simulink model "DvrSimKeybdGD_cs_old"  (R2016a)
settings: Solver=ode5  SolverMode=SingleTasking  StartTime=0.0  StopTime=inf  FixedStep=1/1000  RelTol=1e-3
PreLoadFcn:
  | mbxruntime.callbacks.PreLoadFcn(bdroot);
PostLoadFcn:
  | mbxruntime.callbacks.PostLoadFcn(bdroot);
InitFcn:
  | mbxruntime.callbacks.InitFcn(bdroot);
StartFcn:
  | mbxruntime.callbacks.StartFcn(bdroot);
StopFcn:
  | mbxruntime.callbacks.StopFcn(bdroot);
model workspace (MAT data in the model file):
  mbox_table : struct (value not decoded)
  model_closed = 0
  sim_status = 0
undefined symbols (not defined in the file or in its folder): BMotor1, BMotor2, BrkDelayTime, DControlB, Delay1, Delay2, DiscIntNeverNeededParam, IControlB, JMotor1, JMotor2, PControlB, PreScanCarSimLoadFcn, ratioGearF, ratioGearR, TorqDelayTime, Tstep
undefined symbols (not defined in the file): SteeringColumn, SteeringWheel, WheelL0, WheelL1, WheelR0, WheelR1
libraries: PreScanSimulinkLibrary x35, simulink_extras x26, simulink x26, MyLib x3, Solver_SF x2, pil_lib x1, PreScanUsefulBlocks x1
(part 7 of 12)

== system DvrSimKeybdGD_cs_old/Roewe_550_S_Sedan_1/LaneMarkerSensor_4_Data/If Action Subsystem3 ==
  In1 : Inport
  In2 : Inport  Port=2
  Action Port : ActionPort  ActionType=then
  Bus Selector : BusSelector  OutputSignals=DATA
  Selector : Selector  IndexOptions=Index vector (port)  Indices=[4]  OutputSizes=1
  Out1 : Outport
  wires:
  Bus Selector/1 -> Out1/1  "<DATA>"
  Selector/1 -> Bus Selector/1
  In1/1 -> Selector/1
  In2/1 -> Selector/2

== system DvrSimKeybdGD_cs_old/Roewe_550_S_Sedan_1/LaneMarkerSensor_4_Data/If Action Subsystem4 ==
  In1 : Inport
  In2 : Inport  Port=2
  Action Port : ActionPort  ActionType=then
  Bus Selector : BusSelector  OutputSignals=DATA
  Selector : Selector  IndexOptions=Index vector (port)  Indices=[4]  OutputSizes=1
  Out1 : Outport
  wires:
  Bus Selector/1 -> Out1/1  "<DATA>"
  Selector/1 -> Bus Selector/1
  In1/1 -> Selector/1
  In2/1 -> Selector/2

== system DvrSimKeybdGD_cs_old/Roewe_550_S_Sedan_1/LaneMarkerSensor_5_Data/If Action Subsystem1 ==
  In1 : Inport
  In2 : Inport  Port=2
  Action Port : ActionPort  ActionType=then
  Bus Selector : BusSelector  OutputSignals=DATA
  Selector : Selector  IndexOptions=Index vector (port)  Indices=[4]  OutputSizes=1
  Out1 : Outport
  wires:
  Bus Selector/1 -> Out1/1  "<DATA>"
  Selector/1 -> Bus Selector/1
  In1/1 -> Selector/1
  In2/1 -> Selector/2

== system DvrSimKeybdGD_cs_old/Roewe_550_S_Sedan_1/LaneMarkerSensor_5_Data/If Action Subsystem2 ==
  In1 : Inport
  In2 : Inport  Port=2
  Action Port : ActionPort  ActionType=then
  Bus Selector : BusSelector  OutputSignals=DATA
  Selector : Selector  IndexOptions=Index vector (port)  Indices=[4]  OutputSizes=1
  Out1 : Outport
  wires:
  Bus Selector/1 -> Out1/1  "<DATA>"
  Selector/1 -> Bus Selector/1
  In1/1 -> Selector/1
  In2/1 -> Selector/2

== system DvrSimKeybdGD_cs_old/Roewe_550_S_Sedan_1/LaneMarkerSensor_5_Data/If Action Subsystem3 ==
  In1 : Inport
  In2 : Inport  Port=2
  Action Port : ActionPort  ActionType=then
  Bus Selector : BusSelector  OutputSignals=DATA
  Selector : Selector  IndexOptions=Index vector (port)  Indices=[4]  OutputSizes=1
  Out1 : Outport
  wires:
  Bus Selector/1 -> Out1/1  "<DATA>"
  Selector/1 -> Bus Selector/1
  In1/1 -> Selector/1
  In2/1 -> Selector/2

== system DvrSimKeybdGD_cs_old/Roewe_550_S_Sedan_1/LaneMarkerSensor_5_Data/If Action Subsystem4 ==
  In1 : Inport
  In2 : Inport  Port=2
  Action Port : ActionPort  ActionType=then
  Bus Selector : BusSelector  OutputSignals=DATA
  Selector : Selector  IndexOptions=Index vector (port)  Indices=[4]  OutputSizes=1
  Out1 : Outport
  wires:
  Bus Selector/1 -> Out1/1  "<DATA>"
  Selector/1 -> Bus Selector/1
  In1/1 -> Selector/1
  In2/1 -> Selector/2

== system DvrSimKeybdGD_cs_old/Roewe_550_S_Sedan_1/PreScan_RayCast_Contact_Sensor/Contact Point Bus Creator ==
  demux in : Inport
  Bus Creator : BusCreator  Inputs=3
  Bus Creator1 : BusCreator  Inputs=3
  Bus Creator2 : BusCreator  Inputs=3
  Demux : Demux  Outputs=3
  Demux5 : Demux  Outputs=[3 3 1]
  Demux6 : Demux  Outputs=3
  bus out : Outport
  wires:
  Demux/1 -> Bus Creator/1  "x"
  Demux/2 -> Bus Creator/2  "y"
  Demux/3 -> Bus Creator/3  "z"
  Demux6/1 -> Bus Creator1/1  "x"
  Demux6/2 -> Bus Creator1/2  "y"
  Demux6/3 -> Bus Creator1/3  "z"
  demux in/1 -> Demux5/1
  Demux5/3 -> Bus Creator2/3  "penetrationdepth"
  Bus Creator2/1 -> bus out/1
  Demux5/1 -> Demux/1
  Demux5/2 -> Demux6/1
  Bus Creator/1 -> Bus Creator2/1  "normal"
  Bus Creator1/1 -> Bus Creator2/2  "position"

== system DvrSimKeybdGD_cs_old/Roewe_550_S_Sedan_1/PreScan_RayCast_Contact_Sensor/Contact Point Bus Creator1 ==
  demux in : Inport
  Bus Creator : BusCreator  Inputs=3
  Bus Creator1 : BusCreator  Inputs=3
  Bus Creator2 : BusCreator  Inputs=3
  Demux : Demux  Outputs=3
  Demux5 : Demux  Outputs=[3 3 1]
  Demux6 : Demux  Outputs=3
  bus out : Outport
  wires:
  Bus Creator1/1 -> Bus Creator2/2  "position"
  Bus Creator/1 -> Bus Creator2/1  "normal"
  Demux5/2 -> Demux6/1
  Demux5/1 -> Demux/1
  Bus Creator2/1 -> bus out/1
  Demux5/3 -> Bus Creator2/3  "penetrationdepth"
  demux in/1 -> Demux5/1
  Demux6/3 -> Bus Creator1/3  "z"
  Demux6/2 -> Bus Creator1/2  "y"
  Demux6/1 -> Bus Creator1/1  "x"
  Demux/3 -> Bus Creator/3  "z"
  Demux/2 -> Bus Creator/2  "y"
  Demux/1 -> Bus Creator/1  "x"

== system DvrSimKeybdGD_cs_old/Roewe_550_S_Sedan_1/PreScan_RayCast_Contact_Sensor/Contact Point Bus Creator2 ==
  demux in : Inport
  Bus Creator : BusCreator  Inputs=3
  Bus Creator1 : BusCreator  Inputs=3
  Bus Creator2 : BusCreator  Inputs=3
  Demux : Demux  Outputs=3
  Demux5 : Demux  Outputs=[3 3 1]
  Demux6 : Demux  Outputs=3
  bus out : Outport
  wires:
  Bus Creator1/1 -> Bus Creator2/2  "position"
  Bus Creator/1 -> Bus Creator2/1  "normal"
  Demux5/2 -> Demux6/1
  Demux5/1 -> Demux/1
  Bus Creator2/1 -> bus out/1
  Demux5/3 -> Bus Creator2/3  "penetrationdepth"
  demux in/1 -> Demux5/1
  Demux6/3 -> Bus Creator1/3  "z"
  Demux6/2 -> Bus Creator1/2  "y"
  Demux6/1 -> Bus Creator1/1  "x"
  Demux/3 -> Bus Creator/3  "z"
  Demux/2 -> Bus Creator/2  "y"
  Demux/1 -> Bus Creator/1  "x"

== system DvrSimKeybdGD_cs_old/Roewe_550_S_Sedan_1/PreScan_RayCast_Contact_Sensor/Contact Point Bus Creator3 ==
  demux in : Inport
  Bus Creator : BusCreator  Inputs=3
  Bus Creator1 : BusCreator  Inputs=3
  Bus Creator2 : BusCreator  Inputs=3
  Demux : Demux  Outputs=3
  Demux5 : Demux  Outputs=[3 3 1]
  Demux6 : Demux  Outputs=3
  bus out : Outport
  wires:
  Bus Creator1/1 -> Bus Creator2/2  "position"
  Bus Creator/1 -> Bus Creator2/1  "normal"
  Demux5/2 -> Demux6/1
  Demux5/1 -> Demux/1
  Bus Creator2/1 -> bus out/1
  Demux5/3 -> Bus Creator2/3  "penetrationdepth"
  demux in/1 -> Demux5/1
  Demux6/3 -> Bus Creator1/3  "z"
  Demux6/2 -> Bus Creator1/2  "y"
  Demux6/1 -> Bus Creator1/1  "x"
  Demux/3 -> Bus Creator/3  "z"
  Demux/2 -> Bus Creator/2  "y"
  Demux/1 -> Bus Creator/1  "x"

== system DvrSimKeybdGD_cs_old/Roewe_550_S_Sedan_1/PreScan_RayCast_Contact_Sensor/For All Wheel Contacts ==
  In1 : Inport  Partition=on  PartitionDimension=1  PartitionWidth=1
  Bus Selector : BusSelector  OutputSignals=NORMAL.X,NORMAL.Y,NORMAL.Z,POSITION.X,POSITION.Y,POSITION.Z,PENETRATIONDEPTH
  For Each : ForEach  DisableCoverage=on  IndexMode=One-based
  Mux : Mux  Inputs=7
  Out1 : Outport  ConcatenationDimension=1
  wires:
  In1/1 -> Bus Selector/1
  Bus Selector/1 -> Mux/1  "<X>"
  Bus Selector/2 -> Mux/2  "<Y>"
  Bus Selector/3 -> Mux/3  "<Z>"
  Bus Selector/4 -> Mux/4  "<X>"
  Bus Selector/5 -> Mux/5  "<Y>"
  Bus Selector/6 -> Mux/6  "<Z>"
  Bus Selector/7 -> Mux/7  "<PENETRATIONDEPTH>"
  Mux/1 -> Out1/1

== system DvrSimKeybdGD_cs_old/Roewe_550_S_Sedan_1/PreScan_RayCast_Contact_Sensor/Subsystem1 ==
  In1 : Inport
  sfun_WheelContactsRayCast : S-Function  FunctionName=sfun_WheelContactsRayCast  Parameters=SParameter1, SParameter2, SParameter3, SParameter4, SParameter5, SampleTime  SFunctionDeploymentMode=off  EnableBusSupport=off  mask(Legacy Function){SFunctionSpec=void prescan_outputFcn(void ** work1,  PRESCAN_POSEQ_DATA u1[p3], PRESCAN_WHEELCONTACT_DATA y1[p4]), SParameter1=uint8([fullfile(pwd,'Experiment.pex') 0]), SParameter2=uint8([0 0]), SParameter3=NumberOfWheels, SParameter4=NumberOfWheels*MaxContactPoints, SParameter5=Range, SampleTime=-1, ShowSpec=on}
      mask prompts: SParameter1 "P1:"; SParameter2 "P2:"; SParameter3 "P3:"; SParameter4 "P4:"; SParameter5 "P5:"; SampleTime "Sample time (-1 for inherited):"; ShowSpec "Display function specification"
      mask help:
      | This block allows you to call the legacy functions specified by the following Legacy Code Tool definition:
      | def.SFunctionName = 'sfun_WheelContactsRayCast';
      | def.OutputFcnSpec = 'void prescan_outputFcn(void ** work1,  PRESCAN_POSEQ_DATA u1[p3], PRESCAN_WHEELCONTACT_DATA y1[p4])';
      | def.StartFcnSpec = 'void prescan_startFcn(void ** work1, uint8 p1[], uint8 p2[], double p3, double p4, double p5)';
      | def.TerminateFcnSpec = 'void prescan_terminateFcn(void ** work1)';
      | def.HeaderFiles = {'prescan_wheelcontactsraycast_data.h', 'prescan_header_data.h', 'prescan_SFunLibrary.h', 'prescan_CreateLogHandler.h', 'prescan_CreateErrorHandler.h'};
      | def.SourceFiles = {'prescan_MexLogHandler.cpp', 'prescan_SimStructErrorHandler.cpp', 'prescan_ConcurrentLogHandler.cpp', 'prescan_ConcurrentErrorHandler.cpp'};
      | def.HostLibFiles = {'sensorinterfaced.lib'};
      | def.TargetLibFiles = {'sensorinterfaced.so'};
      | def.IncPaths = {'.', 'C:\prescandev\vislibrary\vis\..\pimp\include\sensors\InterfaceRTW'};
      | def.SrcPaths = {'.'};
      | def.LibPaths = {'C:\\prescandev\\vislibrary_build\lib'};
      | def.SampleTime = 'parameterized';
      mask Help: <p>This block was generated automatically by the Legacy Code Tool. For detailed help on this tool, call<a href="matlab:legacy_code('help')"> legacy_code('help')</a>.</p>
      mask Callback ShowSpec:
      | if strcmp(get_param(gcbh, 'ShowSpec'), 'on')
      |   set_param(gcbh, 'MaskDisplay', sprintf('fprintf(''%s'');', get_param(gcbh, 'SFunctionSpec')));
      | else
      |   set_param(gcbh, 'MaskDisplay', sprintf('fprintf(''%s'');', get_param(gcbh, 'FunctionName')));
      | end
      mask Display: fprintf('void prescan_outputFcn(void ** work1,  PRESCAN_POSEQ_DATA u1[p3], PRESCAN_WHEELCONTACT_DATA y1[p4])');
  Out1 : Outport
  wires:
  In1/1 -> sfun_WheelContactsRayCast/1
  sfun_WheelContactsRayCast/1 -> Out1/1

== system DvrSimKeybdGD_cs_old/Roewe_550_S_Sedan_1/PreScan_RayCast_Contact_Sensor/Subsystem2 ==
  Wheel poses : Inport
  Wheel radius : Inport  Port=2
  Vehicle orientation : Inport  Port=3
  Bus Creator : BusCreator  Inputs=3
  Demux3 : Demux  Outputs=3
  sfun_WheelPoseCorrection : S-Function  FunctionName=sfun_WheelPoseCorrection  Parameters=SParameter1, SampleTime  SFunctionDeploymentMode=off  EnableBusSupport=off  mask(Legacy Function){SFunctionSpec=void prescan_outputFcn(void ** work1,  PRESCAN_POSEQ_DATA u1[p1], double u2[p1], PRESCAN_RPY_DATA u3[1], PRESCAN_POSEQ_DATA y1[p1]), SParameter1=nrOfWheels, SampleTime=-1, ShowSpec=on}
      mask prompts: SParameter1 "P1:"; SampleTime "Sample time (-1 for inherited):"; ShowSpec "Display function specification"
      mask help:
      | This block allows you to call the legacy functions specified by the following Legacy Code Tool definition:
      | def.SFunctionName = 'sfun_WheelPoseCorrection';
      | def.OutputFcnSpec = 'void prescan_outputFcn(void ** work1,  PRESCAN_POSEQ_DATA u1[p1], double u2[p1], PRESCAN_RPY_DATA u3[1], PRESCAN_POSEQ_DATA y1[p1])';
      | def.StartFcnSpec = 'void prescan_startFcn(void ** work1, double p1)';
      | def.TerminateFcnSpec = 'void prescan_terminateFcn(void ** work1)';
      | def.HeaderFiles = {'prescan_wheelposecorrection_data.h', 'prescan_header_data.h', 'prescan_SFunLibrary.h', 'prescan_CreateLogHandler.h', 'prescan_CreateErrorHandler.h'};
      | def.SourceFiles = {'prescan_MexLogHandler.cpp', 'prescan_SimStructErrorHandler.cpp', 'prescan_ConcurrentLogHandler.cpp', 'prescan_ConcurrentErrorHandler.cpp'};
      | def.HostLibFiles = {'sensorinterfaced.lib'};
      | def.TargetLibFiles = {'sensorinterfaced.so'};
      | def.IncPaths = {'.', 'C:\prescandev\vislibrary\vis\..\pimp\include\sensors\InterfaceRTW'};
      | def.SrcPaths = {'.'};
      | def.LibPaths = {'C:\\prescandev\\vislibrary_build\lib'};
      | def.SampleTime = 'parameterized';
      mask Help: <p>This block was generated automatically by the Legacy Code Tool. For detailed help on this tool, call<a href="matlab:legacy_code('help')"> legacy_code('help')</a>.</p>
      mask Callback ShowSpec:
      | if strcmp(get_param(gcbh, 'ShowSpec'), 'on')
      |   set_param(gcbh, 'MaskDisplay', sprintf('fprintf(''%s'');', get_param(gcbh, 'SFunctionSpec')));
      | else
      |   set_param(gcbh, 'MaskDisplay', sprintf('fprintf(''%s'');', get_param(gcbh, 'FunctionName')));
      | end
      mask Display: fprintf('void prescan_outputFcn(void ** work1,  PRESCAN_POSEQ_DATA u1[p1], double u2[p1], PRESCAN_RPY_DATA u3[1], PRESCAN_POSEQ_DATA y1[p1])');
  Virtual Poses : Outport
  wires:
  Demux3/1 -> Bus Creator/1  "Roll"
  Demux3/2 -> Bus Creator/2  "Pitch"
  Demux3/3 -> Bus Creator/3  "Yaw"
  Bus Creator/1 -> sfun_WheelPoseCorrection/3
  Wheel radius/1 -> sfun_WheelPoseCorrection/2
  Vehicle orientation/1 -> Demux3/1
  sfun_WheelPoseCorrection/1 -> Virtual Poses/1
  Wheel poses/1 -> sfun_WheelPoseCorrection/1

== system DvrSimKeybdGD_cs_old/Roewe_550_S_Sedan_1/PreScan_RayCast_Contact_Sensor/Vehicle Local to World ==
  State : Inport
  Demux1 : Demux  Outputs=[3 3]
  iniBODYAngles wrtVEH [rad] : Constant  Value=[Roll0 Pitch0 0]  SampleTime=Inf
  iniVEHAngles wrtGLOB [rad] : Constant  Value=[0 0 Yaw0]  SampleTime=Inf
  iniVEHposition wrtGLOB [m] : Constant  Value=[x0 y0 z0]  SampleTime=Inf
  state2FullState : Subsystem  mask(PreScan Demux Block:){}
  Position : Outport
  Orientation : Outport  Port=2
  wires:
  iniVEHAngles wrtGLOB [rad]/1 -> state2FullState/4(iniVEH Angles wrt GLOB axis system [deg])
  iniBODYAngles wrtVEH [rad]/1 -> state2FullState/3(iniBODY Angles wrt VEH axis system [deg])
  iniVEHposition wrtGLOB [m]/1 -> state2FullState/2(ini VEHpos wrt GLOB axis system [m])
  Demux1/2 -> Orientation/1
  Demux1/1 -> Position/1
  State/1 -> state2FullState/1(dx,dy,dz [m/s] R,P,Y [rad])
  state2FullState/1(State) -> Demux1/1

== system DvrSimKeybdGD_cs_old/Roewe_550_S_Sedan_1/PreScan_RayCast_Contact_Sensor/Wheels = 4 ==
  Vehicle wrt World : Inport
  Wheels wrt World : Inport  Port=2
  Bus Creator : BusCreator  Inputs=3  OutDataTypeStr=Bus: PRESCAN_XYZ_DATA  NonVirtualBus=on
  Bus Creator1 : BusCreator  Inputs=3  OutDataTypeStr=Bus: PRESCAN_RPY_DATA  NonVirtualBus=on
  Bus Creator3 : BusCreator  Inputs=2  OutDataTypeStr=Bus: PRESCAN_POSE_DATA  NonVirtualBus=on
  Demux3 : Demux  Outputs=6
  FL : Selector  InputPortWidth=28  IndexOptions=Index vector (dialog)  Indices=[(1:7)]  OutputSizes=1
  FR : Selector  InputPortWidth=28  IndexOptions=Index vector (dialog)  Indices=[(8:14)]  OutputSizes=1
  RL : Selector  InputPortWidth=28  IndexOptions=Index vector (dialog)  Indices=[(15:21)]  OutputSizes=1
  RR : Selector  InputPortWidth=28  IndexOptions=Index vector (dialog)  Indices=[(22:28)]  OutputSizes=1
  Vector Concatenate1 : Concatenate  NumInputs=4
  sfun_Wheels2World : S-Function  FunctionName=sfun_Wheels2World  Parameters=SParameter1, SParameter2, SParameter3, SampleTime  SFunctionDeploymentMode=off  EnableBusSupport=off  mask(Legacy Function){SFunctionSpec=void prescan_outputFcn(void ** work1,  PRESCAN_POSE_DATA u1[1], PRESCAN_POSEA_DATA u2[p1], PRESCAN_POSEQ_DATA y1[p1]), SParameter1=NumberOfWheels, SParameter2=hcog, SParameter3=b, SampleTime=-1, ShowSpec=on}
      mask prompts: SParameter1 "P1:"; SParameter2 "P2:"; SParameter3 "P3:"; SampleTime "Sample time (-1 for inherited):"; ShowSpec "Display function specification"
      mask help:
      | This block allows you to call the legacy functions specified by the following Legacy Code Tool definition:
      | def.SFunctionName = 'sfun_Wheels2World';
      | def.OutputFcnSpec = 'void prescan_outputFcn(void ** work1,  PRESCAN_POSE_DATA u1[1], PRESCAN_POSEA_DATA u2[p1], PRESCAN_POSEQ_DATA y1[p1])';
      | def.StartFcnSpec = 'void prescan_startFcn(void ** work1, double p1, double p2, double p3)';
      | def.TerminateFcnSpec = 'void prescan_terminateFcn(void ** work1)';
      | def.HeaderFiles = {'prescan_wheels2world_data.h', 'prescan_header_data.h', 'prescan_SFunLibrary.h', 'prescan_CreateLogHandler.h', 'prescan_CreateErrorHandler.h'};
      | def.SourceFiles = {'prescan_MexLogHandler.cpp', 'prescan_SimStructErrorHandler.cpp', 'prescan_ConcurrentLogHandler.cpp', 'prescan_ConcurrentErrorHandler.cpp'};
      | def.HostLibFiles = {'sensorinterfaced.lib'};
      | def.TargetLibFiles = {'sensorinterfaced.so'};
      | def.IncPaths = {'.', 'C:\prescandev\vislibrary\vis\..\pimp\include\sensors\InterfaceRTW'};
      | def.SrcPaths = {'.'};
      | def.LibPaths = {'C:\\prescandev\\vislibrary_build\lib'};
      | def.SampleTime = 'parameterized';
      mask Help: <p>This block was generated automatically by the Legacy Code Tool. For detailed help on this tool, call<a href="matlab:legacy_code('help')"> legacy_code('help')</a>.</p>
      mask Callback ShowSpec:
      | if strcmp(get_param(gcbh, 'ShowSpec'), 'on')
      |   set_param(gcbh, 'MaskDisplay', sprintf('fprintf(''%s'');', get_param(gcbh, 'SFunctionSpec')));
      | else
      |   set_param(gcbh, 'MaskDisplay', sprintf('fprintf(''%s'');', get_param(gcbh, 'FunctionName')));
      | end
      mask Display: fprintf('void prescan_outputFcn(void ** work1,  PRESCAN_POSE_DATA u1[1], PRESCAN_POSEA_DATA u2[p1], PRESCAN_POSEQ_DATA y1[p1])');
  wheelposeFL : Subsystem
  wheelposeFR : Subsystem
  wheelposeRL : Subsystem
  wheelposeRR : Subsystem
  WheelPoses : Outport
  wires:
  FL/1 -> wheelposeFL/1(vector)
  FR/1 -> wheelposeFR/1(vector)
  RL/1 -> wheelposeRL/1(vector)
  RR/1 -> wheelposeRR/1(vector)
  wheelposeFL/1(bus) -> Vector Concatenate1/1
  Demux3/1 -> Bus Creator/1  "X"
  Demux3/2 -> Bus Creator/2  "Y"
  Demux3/3 -> Bus Creator/3  "Z"
  Demux3/4 -> Bus Creator1/1  "Roll"
  Demux3/5 -> Bus Creator1/2  "Pitch"
  Demux3/6 -> Bus Creator1/3  "Yaw"
  Bus Creator/1 -> Bus Creator3/1  "POSITION"
  Bus Creator1/1 -> Bus Creator3/2  "ORIENTATION"
  Vehicle wrt World/1 -> Demux3/1
  Wheels wrt World/1 -> FL/1, FR/1, RL/1, RR/1
  sfun_Wheels2World/1 -> WheelPoses/1
  wheelposeFR/1(bus) -> Vector Concatenate1/2
  wheelposeRL/1(bus) -> Vector Concatenate1/3
  wheelposeRR/1(bus) -> Vector Concatenate1/4
  Bus Creator3/1 -> sfun_Wheels2World/1
  Vector Concatenate1/1 -> sfun_Wheels2World/2

== system DvrSimKeybdGD_cs_old/Roewe_550_S_Sedan_1/PreScan_RayCast_Contact_Sensor/Wheels Local to World ==
  Steer Angle Front [deg] : Inport  SampleTime=TimeStep
  Steer Angle Rear [deg] : Inport  Port=2  SampleTime=TimeStep
  Velocity [m/s] : Inport  Port=3  SampleTime=TimeStep
  Disp FL [m] : Inport  Port=4  SampleTime=TimeStep
  Disp FR [m] : Inport  Port=5  SampleTime=TimeStep
  Disp RL [m] : Inport  Port=6  SampleTime=TimeStep
  Disp RR [m] : Inport  Port=7  SampleTime=TimeStep
  Constant{4..7} (4 alike) : Constant  Value=0  SampleTime=Inf
  Discrete-Time Integrator : DiscreteIntegrator  SampleTime=TimeStep  ICPrevOutput=DiscIntNeverNeededParam  ICPrevScaledInput=DiscIntNeverNeededParam
  Mux{,1..3} (4 alike) : Mux  Inputs=3
  Mux5 : Mux  Inputs=[3 4 3 4 3 4 3 4]
  Radians to Degrees : simulink_extras/Transformations/Radians to Degrees
  Saturation{,2,4,6} (4 alike) : Saturate  UpperLimit=[0.2 0.2 0.5]  LowerLimit=[-0.2 -0.2 -0.5]
  Saturation{1,3,5,8} (4 alike) : Saturate  UpperLimit=[30 inf 30]  LowerLimit=[-30 -inf -30]
  conv_RotWheelFL : Subsystem
  conv_RotWheelFR : Subsystem
  conv_RotWheelRL : Subsystem
  conv_RotWheelRR : Subsystem
  conv_TransWheelFL : Subsystem  mask(Translation node configuration){tp=Front-Left Wheel, gains=off, Gain_xISO=1, Gain_yISO=1, Gain_zISO=1}
      mask prompts: tp "Type"; gains "Edit scaling factors?"; Gain_xISO "Scaling factor in x-direction (ISO-convention)"; Gain_yISO "Scaling factor in y-direction (ISO-convention)"; Gain_zISO "Scaling factor in z-direction (ISO-convention)"
      mask init:
      | x_ini_VRML = 2.701790; 
      | y_ini_VRML = 0.665750; 
      | z_ini_VRML = 0.317714;
      mask TypeOptions tp: Front-Left Wheel | Front-Right Wheel | Rear-Left Wheel | Rear-Right Wheel | Left Seat | Right Seat
      mask Callback gains:
      | if strcmp(get_param(gcb, 'gains'),'on')
      |     set_param(gcb,'MaskVisibilities',{'on','on','on','on','on'})
      | else
      |     set_param(gcb,'MaskVisibilities',{'on','on','off','off','off'})
      | end
  conv_TransWheelFR : Subsystem  mask(Translation node configuration){tp=Front-Right Wheel, gains=off, Gain_xISO=1, Gain_yISO=1, Gain_zISO=1}
      mask prompts: tp "Type"; gains "Edit scaling factors?"; Gain_xISO "Scaling factor in x-direction (ISO-convention)"; Gain_yISO "Scaling factor in y-direction (ISO-convention)"; Gain_zISO "Scaling factor in z-direction (ISO-convention)"
      mask init:
      | x_ini_VRML = 2.701790; 
      | y_ini_VRML = -0.665750; 
      | z_ini_VRML = 0.317714;
      mask TypeOptions tp: Front-Left Wheel | Front-Right Wheel | Rear-Left Wheel | Rear-Right Wheel | Left Seat | Right Seat
      mask Callback gains:
      | if strcmp(get_param(gcb, 'gains'),'on')
      |     set_param(gcb,'MaskVisibilities',{'on','on','on','on','on'})
      | else
      |     set_param(gcb,'MaskVisibilities',{'on','on','off','off','off'})
      | end
  conv_TransWheelRL : Subsystem  mask(Translation node configuration){tp=Rear-Left Wheel, gains=off, Gain_xISO=1, Gain_yISO=1, Gain_zISO=1}
      mask prompts: tp "Type"; gains "Edit scaling factors?"; Gain_xISO "Scaling factor in x-direction (ISO-convention)"; Gain_yISO "Scaling factor in y-direction (ISO-convention)"; Gain_zISO "Scaling factor in z-direction (ISO-convention)"
      mask init:
      | x_ini_VRML = 0.000000; 
      | y_ini_VRML = 0.665750; 
      | z_ini_VRML = 0.317714;
      mask TypeOptions tp: Front-Left Wheel | Front-Right Wheel | Rear-Left Wheel | Rear-Right Wheel | Left Seat | Right Seat
      mask Callback gains:
      | if strcmp(get_param(gcb, 'gains'),'on')
      |     set_param(gcb,'MaskVisibilities',{'on','on','on','on','on'})
      | else
      |     set_param(gcb,'MaskVisibilities',{'on','on','off','off','off'})
      | end
  conv_TransWheelRR : Subsystem  mask(Translation node configuration){tp=Rear-Right Wheel, gains=off, Gain_xISO=1, Gain_yISO=1, Gain_zISO=1}
      mask prompts: tp "Type"; gains "Edit scaling factors?"; Gain_xISO "Scaling factor in x-direction (ISO-convention)"; Gain_yISO "Scaling factor in y-direction (ISO-convention)"; Gain_zISO "Scaling factor in z-direction (ISO-convention)"
      mask init:
      | x_ini_VRML = 0.000000; 
      | y_ini_VRML = -0.665750; 
      | z_ini_VRML = 0.317714;
      mask TypeOptions tp: Front-Left Wheel | Front-Right Wheel | Rear-Left Wheel | Rear-Right Wheel | Left Seat | Right Seat
      mask Callback gains:
      | if strcmp(get_param(gcb, 'gains'),'on')
      |     set_param(gcb,'MaskVisibilities',{'on','on','on','on','on'})
      | else
      |     set_param(gcb,'MaskVisibilities',{'on','on','off','off','off'})
      | end
  omega=V/Rwheel : Gain  Gain=1/0.29
  Wheel Poses : Outport
  wires:
  conv_RotWheelRR/1(QuaternionVisu [rad]) -> Mux5/8
  conv_RotWheelRL/1(QuaternionVisu [rad]) -> Mux5/6
  conv_TransWheelRR/1(transVisu [m]) -> Mux5/7
  conv_TransWheelRL/1(transVisu [m]) -> Mux5/5
  conv_RotWheelFR/1(QuaternionVisu [rad]) -> Mux5/4
  conv_TransWheelFR/1(transVisu [m]) -> Mux5/3
  conv_RotWheelFL/1(QuaternionVisu [rad]) -> Mux5/2
  conv_TransWheelFL/1(transVisu [m]) -> Mux5/1
  Saturation/1 -> conv_TransWheelFL/1(transISO [m])
  Saturation8/1 -> conv_RotWheelFL/1(BryantISO [deg])
  Saturation2/1 -> conv_TransWheelFR/1(transISO [m])
  Saturation1/1 -> conv_RotWheelFR/1(BryantISO [deg])
  Saturation4/1 -> conv_TransWheelRL/1(transISO [m])
  Saturation3/1 -> conv_RotWheelRL/1(BryantISO [deg])
  Saturation6/1 -> conv_TransWheelRR/1(transISO [m])
  Saturation5/1 -> conv_RotWheelRR/1(BryantISO [deg])
  Mux5/1 -> Wheel Poses/1
  Mux2/1 -> Saturation3/1  "xyz rotation RL [deg]"
  Mux3/1 -> Saturation5/1  "xyz rotation RR [deg]"
  Mux/1 -> Saturation8/1  "xyz rotation FL [deg]"
  Mux1/1 -> Saturation1/1  "xyz rotation FR [deg]"
  Velocity [m/s]/1 -> omega=V/Rwheel/1
  omega=V/Rwheel/1 -> Radians to Degrees/1  "rotational speed [rad/s]"
  Steer Angle Rear [deg]/1 -> Mux2/3, Mux3/3  "rotz"
  Steer Angle Front [deg]/1 -> Mux/3, Mux1/3  "rotz"
  Constant4/1 -> Mux/1  "rotx"
  Constant5/1 -> Mux1/1  "rotx"
  Constant6/1 -> Mux2/1  "rotx"
  Constant7/1 -> Mux3/1  "rotx"
  Radians to Degrees/1 -> Discrete-Time Integrator/1
  Discrete-Time Integrator/1 -> Mux3/2, Mux2/2, Mux1/2, Mux/2  "roty"
  Disp FL [m]/1 -> Saturation/1
  Disp FR [m]/1 -> Saturation2/1
  Disp RL [m]/1 -> Saturation4/1
  Disp RR [m]/1 -> Saturation6/1

== system DvrSimKeybdGD_cs_old/Roewe_550_S_Sedan_1/PreScan_RayCast_Contact_Sensor1/Contact Point Bus Creator ==
  demux in : Inport
  Bus Creator : BusCreator  Inputs=3
  Bus Creator1 : BusCreator  Inputs=3
  Bus Creator2 : BusCreator  Inputs=3
  Demux : Demux  Outputs=3
  Demux5 : Demux  Outputs=[3 3 1]
  Demux6 : Demux  Outputs=3
  bus out : Outport
  wires:
  Demux/1 -> Bus Creator/1  "x"
  Demux/2 -> Bus Creator/2  "y"
  Demux/3 -> Bus Creator/3  "z"
  Demux6/1 -> Bus Creator1/1  "x"
  Demux6/2 -> Bus Creator1/2  "y"
  Demux6/3 -> Bus Creator1/3  "z"
  demux in/1 -> Demux5/1
  Demux5/3 -> Bus Creator2/3  "penetrationdepth"
  Bus Creator2/1 -> bus out/1
  Demux5/1 -> Demux/1
  Demux5/2 -> Demux6/1
  Bus Creator/1 -> Bus Creator2/1  "normal"
  Bus Creator1/1 -> Bus Creator2/2  "position"

== system DvrSimKeybdGD_cs_old/Roewe_550_S_Sedan_1/PreScan_RayCast_Contact_Sensor1/Contact Point Bus Creator1 ==
  demux in : Inport
  Bus Creator : BusCreator  Inputs=3
  Bus Creator1 : BusCreator  Inputs=3
  Bus Creator2 : BusCreator  Inputs=3
  Demux : Demux  Outputs=3
  Demux5 : Demux  Outputs=[3 3 1]
  Demux6 : Demux  Outputs=3
  bus out : Outport
  wires:
  Bus Creator1/1 -> Bus Creator2/2  "position"
  Bus Creator/1 -> Bus Creator2/1  "normal"
  Demux5/2 -> Demux6/1
  Demux5/1 -> Demux/1
  Bus Creator2/1 -> bus out/1
  Demux5/3 -> Bus Creator2/3  "penetrationdepth"
  demux in/1 -> Demux5/1
  Demux6/3 -> Bus Creator1/3  "z"
  Demux6/2 -> Bus Creator1/2  "y"
  Demux6/1 -> Bus Creator1/1  "x"
  Demux/3 -> Bus Creator/3  "z"
  Demux/2 -> Bus Creator/2  "y"
  Demux/1 -> Bus Creator/1  "x"

== system DvrSimKeybdGD_cs_old/Roewe_550_S_Sedan_1/PreScan_RayCast_Contact_Sensor1/Contact Point Bus Creator2 ==
  demux in : Inport
  Bus Creator : BusCreator  Inputs=3
  Bus Creator1 : BusCreator  Inputs=3
  Bus Creator2 : BusCreator  Inputs=3
  Demux : Demux  Outputs=3
  Demux5 : Demux  Outputs=[3 3 1]
  Demux6 : Demux  Outputs=3
  bus out : Outport
  wires:
  Bus Creator1/1 -> Bus Creator2/2  "position"
  Bus Creator/1 -> Bus Creator2/1  "normal"
  Demux5/2 -> Demux6/1
  Demux5/1 -> Demux/1
  Bus Creator2/1 -> bus out/1
  Demux5/3 -> Bus Creator2/3  "penetrationdepth"
  demux in/1 -> Demux5/1
  Demux6/3 -> Bus Creator1/3  "z"
  Demux6/2 -> Bus Creator1/2  "y"
  Demux6/1 -> Bus Creator1/1  "x"
  Demux/3 -> Bus Creator/3  "z"
  Demux/2 -> Bus Creator/2  "y"
  Demux/1 -> Bus Creator/1  "x"

== system DvrSimKeybdGD_cs_old/Roewe_550_S_Sedan_1/PreScan_RayCast_Contact_Sensor1/Contact Point Bus Creator3 ==
  demux in : Inport
  Bus Creator : BusCreator  Inputs=3
  Bus Creator1 : BusCreator  Inputs=3
  Bus Creator2 : BusCreator  Inputs=3
  Demux : Demux  Outputs=3
  Demux5 : Demux  Outputs=[3 3 1]
  Demux6 : Demux  Outputs=3
  bus out : Outport
  wires:
  Bus Creator1/1 -> Bus Creator2/2  "position"
  Bus Creator/1 -> Bus Creator2/1  "normal"
  Demux5/2 -> Demux6/1
  Demux5/1 -> Demux/1
  Bus Creator2/1 -> bus out/1
  Demux5/3 -> Bus Creator2/3  "penetrationdepth"
  demux in/1 -> Demux5/1
  Demux6/3 -> Bus Creator1/3  "z"
  Demux6/2 -> Bus Creator1/2  "y"
  Demux6/1 -> Bus Creator1/1  "x"
  Demux/3 -> Bus Creator/3  "z"
  Demux/2 -> Bus Creator/2  "y"
  Demux/1 -> Bus Creator/1  "x"

== system DvrSimKeybdGD_cs_old/Roewe_550_S_Sedan_1/PreScan_RayCast_Contact_Sensor1/For All Wheel Contacts ==
  In1 : Inport  Partition=on  PartitionDimension=1  PartitionWidth=1
  Bus Selector : BusSelector  OutputSignals=NORMAL.X,NORMAL.Y,NORMAL.Z,POSITION.X,POSITION.Y,POSITION.Z,PENETRATIONDEPTH
  For Each : ForEach  DisableCoverage=on  IndexMode=One-based
  Mux : Mux  Inputs=7
  Out1 : Outport  ConcatenationDimension=1
  wires:
  In1/1 -> Bus Selector/1
  Bus Selector/1 -> Mux/1  "<X>"
  Bus Selector/2 -> Mux/2  "<Y>"
  Bus Selector/3 -> Mux/3  "<Z>"
  Bus Selector/4 -> Mux/4  "<X>"
  Bus Selector/5 -> Mux/5  "<Y>"
  Bus Selector/6 -> Mux/6  "<Z>"
  Bus Selector/7 -> Mux/7  "<PENETRATIONDEPTH>"
  Mux/1 -> Out1/1

== system DvrSimKeybdGD_cs_old/Roewe_550_S_Sedan_1/PreScan_RayCast_Contact_Sensor1/Subsystem1 ==
  In1 : Inport
  sfun_WheelContactsRayCast : S-Function  FunctionName=sfun_WheelContactsRayCast  Parameters=SParameter1, SParameter2, SParameter3, SParameter4, SParameter5, SampleTime  SFunctionDeploymentMode=off  EnableBusSupport=off  mask(Legacy Function){SFunctionSpec=void prescan_outputFcn(void ** work1,  PRESCAN_POSEQ_DATA u1[p3], PRESCAN_WHEELCONTACT_DATA y1[p4]), SParameter1=uint8([fullfile(pwd,'Experiment.pex') 0]), SParameter2=uint8([0 0]), SParameter3=NumberOfWheels, SParameter4=NumberOfWheels*MaxContactPoints, SParameter5=Range, SampleTime=-1, ShowSpec=on}
      mask prompts: SParameter1 "P1:"; SParameter2 "P2:"; SParameter3 "P3:"; SParameter4 "P4:"; SParameter5 "P5:"; SampleTime "Sample time (-1 for inherited):"; ShowSpec "Display function specification"
      mask help:
      | This block allows you to call the legacy functions specified by the following Legacy Code Tool definition:
      | def.SFunctionName = 'sfun_WheelContactsRayCast';
      | def.OutputFcnSpec = 'void prescan_outputFcn(void ** work1,  PRESCAN_POSEQ_DATA u1[p3], PRESCAN_WHEELCONTACT_DATA y1[p4])';
      | def.StartFcnSpec = 'void prescan_startFcn(void ** work1, uint8 p1[], uint8 p2[], double p3, double p4, double p5)';
      | def.TerminateFcnSpec = 'void prescan_terminateFcn(void ** work1)';
      | def.HeaderFiles = {'prescan_wheelcontactsraycast_data.h', 'prescan_header_data.h', 'prescan_SFunLibrary.h', 'prescan_CreateLogHandler.h', 'prescan_CreateErrorHandler.h'};
      | def.SourceFiles = {'prescan_MexLogHandler.cpp', 'prescan_SimStructErrorHandler.cpp', 'prescan_ConcurrentLogHandler.cpp', 'prescan_ConcurrentErrorHandler.cpp'};
      | def.HostLibFiles = {'sensorinterfaced.lib'};
      | def.TargetLibFiles = {'sensorinterfaced.so'};
      | def.IncPaths = {'.', 'C:\prescandev\vislibrary\vis\..\pimp\include\sensors\InterfaceRTW'};
      | def.SrcPaths = {'.'};
      | def.LibPaths = {'C:\\prescandev\\vislibrary_build\lib'};
      | def.SampleTime = 'parameterized';
      mask Help: <p>This block was generated automatically by the Legacy Code Tool. For detailed help on this tool, call<a href="matlab:legacy_code('help')"> legacy_code('help')</a>.</p>
      mask Callback ShowSpec:
      | if strcmp(get_param(gcbh, 'ShowSpec'), 'on')
      |   set_param(gcbh, 'MaskDisplay', sprintf('fprintf(''%s'');', get_param(gcbh, 'SFunctionSpec')));
      | else
      |   set_param(gcbh, 'MaskDisplay', sprintf('fprintf(''%s'');', get_param(gcbh, 'FunctionName')));
      | end
      mask Display: fprintf('void prescan_outputFcn(void ** work1,  PRESCAN_POSEQ_DATA u1[p3], PRESCAN_WHEELCONTACT_DATA y1[p4])');
  Out1 : Outport
  wires:
  In1/1 -> sfun_WheelContactsRayCast/1
  sfun_WheelContactsRayCast/1 -> Out1/1

== system DvrSimKeybdGD_cs_old/Roewe_550_S_Sedan_1/PreScan_RayCast_Contact_Sensor1/Subsystem2 ==
  Wheel poses : Inport
  Wheel radius : Inport  Port=2
  Vehicle orientation : Inport  Port=3
  Bus Creator : BusCreator  Inputs=3
  Demux3 : Demux  Outputs=3
  sfun_WheelPoseCorrection : S-Function  FunctionName=sfun_WheelPoseCorrection  Parameters=SParameter1, SampleTime  SFunctionDeploymentMode=off  EnableBusSupport=off  mask(Legacy Function){SFunctionSpec=void prescan_outputFcn(void ** work1,  PRESCAN_POSEQ_DATA u1[p1], double u2[p1], PRESCAN_RPY_DATA u3[1], PRESCAN_POSEQ_DATA y1[p1]), SParameter1=nrOfWheels, SampleTime=-1, ShowSpec=on}
      mask prompts: SParameter1 "P1:"; SampleTime "Sample time (-1 for inherited):"; ShowSpec "Display function specification"
      mask help:
      | This block allows you to call the legacy functions specified by the following Legacy Code Tool definition:
      | def.SFunctionName = 'sfun_WheelPoseCorrection';
      | def.OutputFcnSpec = 'void prescan_outputFcn(void ** work1,  PRESCAN_POSEQ_DATA u1[p1], double u2[p1], PRESCAN_RPY_DATA u3[1], PRESCAN_POSEQ_DATA y1[p1])';
      | def.StartFcnSpec = 'void prescan_startFcn(void ** work1, double p1)';
      | def.TerminateFcnSpec = 'void prescan_terminateFcn(void ** work1)';
      | def.HeaderFiles = {'prescan_wheelposecorrection_data.h', 'prescan_header_data.h', 'prescan_SFunLibrary.h', 'prescan_CreateLogHandler.h', 'prescan_CreateErrorHandler.h'};
      | def.SourceFiles = {'prescan_MexLogHandler.cpp', 'prescan_SimStructErrorHandler.cpp', 'prescan_ConcurrentLogHandler.cpp', 'prescan_ConcurrentErrorHandler.cpp'};
      | def.HostLibFiles = {'sensorinterfaced.lib'};
      | def.TargetLibFiles = {'sensorinterfaced.so'};
      | def.IncPaths = {'.', 'C:\prescandev\vislibrary\vis\..\pimp\include\sensors\InterfaceRTW'};
      | def.SrcPaths = {'.'};
      | def.LibPaths = {'C:\\prescandev\\vislibrary_build\lib'};
      | def.SampleTime = 'parameterized';
      mask Help: <p>This block was generated automatically by the Legacy Code Tool. For detailed help on this tool, call<a href="matlab:legacy_code('help')"> legacy_code('help')</a>.</p>
      mask Callback ShowSpec:
      | if strcmp(get_param(gcbh, 'ShowSpec'), 'on')
      |   set_param(gcbh, 'MaskDisplay', sprintf('fprintf(''%s'');', get_param(gcbh, 'SFunctionSpec')));
      | else
      |   set_param(gcbh, 'MaskDisplay', sprintf('fprintf(''%s'');', get_param(gcbh, 'FunctionName')));
      | end
      mask Display: fprintf('void prescan_outputFcn(void ** work1,  PRESCAN_POSEQ_DATA u1[p1], double u2[p1], PRESCAN_RPY_DATA u3[1], PRESCAN_POSEQ_DATA y1[p1])');
  Virtual Poses : Outport
  wires:
  Demux3/1 -> Bus Creator/1  "Roll"
  Demux3/2 -> Bus Creator/2  "Pitch"
  Demux3/3 -> Bus Creator/3  "Yaw"
  Bus Creator/1 -> sfun_WheelPoseCorrection/3
  Wheel radius/1 -> sfun_WheelPoseCorrection/2
  Vehicle orientation/1 -> Demux3/1
  sfun_WheelPoseCorrection/1 -> Virtual Poses/1
  Wheel poses/1 -> sfun_WheelPoseCorrection/1

== system DvrSimKeybdGD_cs_old/Roewe_550_S_Sedan_1/PreScan_RayCast_Contact_Sensor1/Vehicle Local to World ==
  State : Inport
  Demux1 : Demux  Outputs=[3 3]
  iniBODYAngles wrtVEH [rad] : Constant  Value=[Roll0 Pitch0 0]  SampleTime=Inf
  iniVEHAngles wrtGLOB [rad] : Constant  Value=[0 0 Yaw0]  SampleTime=Inf
  iniVEHposition wrtGLOB [m] : Constant  Value=[x0 y0 z0]  SampleTime=Inf
  state2FullState : Subsystem  mask(PreScan Demux Block:){}
  Position : Outport
  Orientation : Outport  Port=2
  wires:
  iniVEHAngles wrtGLOB [rad]/1 -> state2FullState/4(iniVEH Angles wrt GLOB axis system [deg])
  iniBODYAngles wrtVEH [rad]/1 -> state2FullState/3(iniBODY Angles wrt VEH axis system [deg])
  iniVEHposition wrtGLOB [m]/1 -> state2FullState/2(ini VEHpos wrt GLOB axis system [m])
  Demux1/2 -> Orientation/1
  Demux1/1 -> Position/1
  State/1 -> state2FullState/1(dx,dy,dz [m/s] R,P,Y [rad])
  state2FullState/1(State) -> Demux1/1

== system DvrSimKeybdGD_cs_old/Roewe_550_S_Sedan_1/PreScan_RayCast_Contact_Sensor1/Wheels = 4 ==
  Vehicle wrt World : Inport
  Wheels wrt World : Inport  Port=2
  Bus Creator : BusCreator  Inputs=3  OutDataTypeStr=Bus: PRESCAN_XYZ_DATA  NonVirtualBus=on
  Bus Creator1 : BusCreator  Inputs=3  OutDataTypeStr=Bus: PRESCAN_RPY_DATA  NonVirtualBus=on
  Bus Creator3 : BusCreator  Inputs=2  OutDataTypeStr=Bus: PRESCAN_POSE_DATA  NonVirtualBus=on
  Demux3 : Demux  Outputs=6
  FL : Selector  InputPortWidth=28  IndexOptions=Index vector (dialog)  Indices=[(1:7)]  OutputSizes=1
  FR : Selector  InputPortWidth=28  IndexOptions=Index vector (dialog)  Indices=[(8:14)]  OutputSizes=1
  RL : Selector  InputPortWidth=28  IndexOptions=Index vector (dialog)  Indices=[(15:21)]  OutputSizes=1
  RR : Selector  InputPortWidth=28  IndexOptions=Index vector (dialog)  Indices=[(22:28)]  OutputSizes=1
  Vector Concatenate1 : Concatenate  NumInputs=4
  sfun_Wheels2World : S-Function  FunctionName=sfun_Wheels2World  Parameters=SParameter1, SParameter2, SParameter3, SampleTime  SFunctionDeploymentMode=off  EnableBusSupport=off  mask(Legacy Function){SFunctionSpec=void prescan_outputFcn(void ** work1,  PRESCAN_POSE_DATA u1[1], PRESCAN_POSEA_DATA u2[p1], PRESCAN_POSEQ_DATA y1[p1]), SParameter1=NumberOfWheels, SParameter2=hcog, SParameter3=b, SampleTime=-1, ShowSpec=on}
      mask prompts: SParameter1 "P1:"; SParameter2 "P2:"; SParameter3 "P3:"; SampleTime "Sample time (-1 for inherited):"; ShowSpec "Display function specification"
      mask help:
      | This block allows you to call the legacy functions specified by the following Legacy Code Tool definition:
      | def.SFunctionName = 'sfun_Wheels2World';
      | def.OutputFcnSpec = 'void prescan_outputFcn(void ** work1,  PRESCAN_POSE_DATA u1[1], PRESCAN_POSEA_DATA u2[p1], PRESCAN_POSEQ_DATA y1[p1])';
      | def.StartFcnSpec = 'void prescan_startFcn(void ** work1, double p1, double p2, double p3)';
      | def.TerminateFcnSpec = 'void prescan_terminateFcn(void ** work1)';
      | def.HeaderFiles = {'prescan_wheels2world_data.h', 'prescan_header_data.h', 'prescan_SFunLibrary.h', 'prescan_CreateLogHandler.h', 'prescan_CreateErrorHandler.h'};
      | def.SourceFiles = {'prescan_MexLogHandler.cpp', 'prescan_SimStructErrorHandler.cpp', 'prescan_ConcurrentLogHandler.cpp', 'prescan_ConcurrentErrorHandler.cpp'};
      | def.HostLibFiles = {'sensorinterfaced.lib'};
      | def.TargetLibFiles = {'sensorinterfaced.so'};
      | def.IncPaths = {'.', 'C:\prescandev\vislibrary\vis\..\pimp\include\sensors\InterfaceRTW'};
      | def.SrcPaths = {'.'};
      | def.LibPaths = {'C:\\prescandev\\vislibrary_build\lib'};
      | def.SampleTime = 'parameterized';
      mask Help: <p>This block was generated automatically by the Legacy Code Tool. For detailed help on this tool, call<a href="matlab:legacy_code('help')"> legacy_code('help')</a>.</p>
      mask Callback ShowSpec:
      | if strcmp(get_param(gcbh, 'ShowSpec'), 'on')
      |   set_param(gcbh, 'MaskDisplay', sprintf('fprintf(''%s'');', get_param(gcbh, 'SFunctionSpec')));
      | else
      |   set_param(gcbh, 'MaskDisplay', sprintf('fprintf(''%s'');', get_param(gcbh, 'FunctionName')));
      | end
      mask Display: fprintf('void prescan_outputFcn(void ** work1,  PRESCAN_POSE_DATA u1[1], PRESCAN_POSEA_DATA u2[p1], PRESCAN_POSEQ_DATA y1[p1])');
  wheelposeFL : Subsystem
  wheelposeFR : Subsystem
  wheelposeRL : Subsystem
  wheelposeRR : Subsystem
  WheelPoses : Outport
  wires:
  FL/1 -> wheelposeFL/1(vector)
  FR/1 -> wheelposeFR/1(vector)
  RL/1 -> wheelposeRL/1(vector)
  RR/1 -> wheelposeRR/1(vector)
  wheelposeFL/1(bus) -> Vector Concatenate1/1
  Demux3/1 -> Bus Creator/1  "X"
  Demux3/2 -> Bus Creator/2  "Y"
  Demux3/3 -> Bus Creator/3  "Z"
  Demux3/4 -> Bus Creator1/1  "Roll"
  Demux3/5 -> Bus Creator1/2  "Pitch"
  Demux3/6 -> Bus Creator1/3  "Yaw"
  Bus Creator/1 -> Bus Creator3/1  "POSITION"
  Bus Creator1/1 -> Bus Creator3/2  "ORIENTATION"
  Vehicle wrt World/1 -> Demux3/1
  Wheels wrt World/1 -> FL/1, FR/1, RL/1, RR/1
  sfun_Wheels2World/1 -> WheelPoses/1
  wheelposeFR/1(bus) -> Vector Concatenate1/2
  wheelposeRL/1(bus) -> Vector Concatenate1/3
  wheelposeRR/1(bus) -> Vector Concatenate1/4
  Bus Creator3/1 -> sfun_Wheels2World/1
  Vector Concatenate1/1 -> sfun_Wheels2World/2

== system DvrSimKeybdGD_cs_old/Roewe_550_S_Sedan_1/PreScan_RayCast_Contact_Sensor1/Wheels Local to World ==
  Steer Angle Front [deg] : Inport  SampleTime=TimeStep
  Steer Angle Rear [deg] : Inport  Port=2  SampleTime=TimeStep
  Velocity [m/s] : Inport  Port=3  SampleTime=TimeStep
  Disp FL [m] : Inport  Port=4  SampleTime=TimeStep
  Disp FR [m] : Inport  Port=5  SampleTime=TimeStep
  Disp RL [m] : Inport  Port=6  SampleTime=TimeStep
  Disp RR [m] : Inport  Port=7  SampleTime=TimeStep
  Constant{4..7} (4 alike) : Constant  Value=0  SampleTime=Inf
  Discrete-Time Integrator : DiscreteIntegrator  SampleTime=TimeStep  ICPrevOutput=DiscIntNeverNeededParam  ICPrevScaledInput=DiscIntNeverNeededParam
  Mux{,1..3} (4 alike) : Mux  Inputs=3
  Mux5 : Mux  Inputs=[3 4 3 4 3 4 3 4]
  Radians to Degrees : simulink_extras/Transformations/Radians to Degrees
  Saturation{,2,4,6} (4 alike) : Saturate  UpperLimit=[0.2 0.2 0.5]  LowerLimit=[-0.2 -0.2 -0.5]
  Saturation{1,3,5,8} (4 alike) : Saturate  UpperLimit=[30 inf 30]  LowerLimit=[-30 -inf -30]
  conv_RotWheelFL : Subsystem
  conv_RotWheelFR : Subsystem
  conv_RotWheelRL : Subsystem
  conv_RotWheelRR : Subsystem
  conv_TransWheelFL : Subsystem  mask(Translation node configuration){tp=Front-Left Wheel, gains=off, Gain_xISO=1, Gain_yISO=1, Gain_zISO=1}
      mask prompts: tp "Type"; gains "Edit scaling factors?"; Gain_xISO "Scaling factor in x-direction (ISO-convention)"; Gain_yISO "Scaling factor in y-direction (ISO-convention)"; Gain_zISO "Scaling factor in z-direction (ISO-convention)"
      mask init:
      | x_ini_VRML = 2.701790; 
      | y_ini_VRML = 0.665750; 
      | z_ini_VRML = 0.317714;
      mask TypeOptions tp: Front-Left Wheel | Front-Right Wheel | Rear-Left Wheel | Rear-Right Wheel | Left Seat | Right Seat
      mask Callback gains:
      | if strcmp(get_param(gcb, 'gains'),'on')
      |     set_param(gcb,'MaskVisibilities',{'on','on','on','on','on'})
      | else
      |     set_param(gcb,'MaskVisibilities',{'on','on','off','off','off'})
      | end
  conv_TransWheelFR : Subsystem  mask(Translation node configuration){tp=Front-Right Wheel, gains=off, Gain_xISO=1, Gain_yISO=1, Gain_zISO=1}
      mask prompts: tp "Type"; gains "Edit scaling factors?"; Gain_xISO "Scaling factor in x-direction (ISO-convention)"; Gain_yISO "Scaling factor in y-direction (ISO-convention)"; Gain_zISO "Scaling factor in z-direction (ISO-convention)"
      mask init:
      | x_ini_VRML = 2.701790; 
      | y_ini_VRML = -0.665750; 
      | z_ini_VRML = 0.317714;
      mask TypeOptions tp: Front-Left Wheel | Front-Right Wheel | Rear-Left Wheel | Rear-Right Wheel | Left Seat | Right Seat
      mask Callback gains:
      | if strcmp(get_param(gcb, 'gains'),'on')
      |     set_param(gcb,'MaskVisibilities',{'on','on','on','on','on'})
      | else
      |     set_param(gcb,'MaskVisibilities',{'on','on','off','off','off'})
      | end
  conv_TransWheelRL : Subsystem  mask(Translation node configuration){tp=Rear-Left Wheel, gains=off, Gain_xISO=1, Gain_yISO=1, Gain_zISO=1}
      mask prompts: tp "Type"; gains "Edit scaling factors?"; Gain_xISO "Scaling factor in x-direction (ISO-convention)"; Gain_yISO "Scaling factor in y-direction (ISO-convention)"; Gain_zISO "Scaling factor in z-direction (ISO-convention)"
      mask init:
      | x_ini_VRML = 0.000000; 
      | y_ini_VRML = 0.665750; 
      | z_ini_VRML = 0.317714;
      mask TypeOptions tp: Front-Left Wheel | Front-Right Wheel | Rear-Left Wheel | Rear-Right Wheel | Left Seat | Right Seat
      mask Callback gains:
      | if strcmp(get_param(gcb, 'gains'),'on')
      |     set_param(gcb,'MaskVisibilities',{'on','on','on','on','on'})
      | else
      |     set_param(gcb,'MaskVisibilities',{'on','on','off','off','off'})
      | end
  conv_TransWheelRR : Subsystem  mask(Translation node configuration){tp=Rear-Right Wheel, gains=off, Gain_xISO=1, Gain_yISO=1, Gain_zISO=1}
      mask prompts: tp "Type"; gains "Edit scaling factors?"; Gain_xISO "Scaling factor in x-direction (ISO-convention)"; Gain_yISO "Scaling factor in y-direction (ISO-convention)"; Gain_zISO "Scaling factor in z-direction (ISO-convention)"
      mask init:
      | x_ini_VRML = 0.000000; 
      | y_ini_VRML = -0.665750; 
      | z_ini_VRML = 0.317714;
      mask TypeOptions tp: Front-Left Wheel | Front-Right Wheel | Rear-Left Wheel | Rear-Right Wheel | Left Seat | Right Seat
      mask Callback gains:
      | if strcmp(get_param(gcb, 'gains'),'on')
      |     set_param(gcb,'MaskVisibilities',{'on','on','on','on','on'})
      | else
      |     set_param(gcb,'MaskVisibilities',{'on','on','off','off','off'})
      | end
  omega=V/Rwheel : Gain  Gain=1/0.29
  Wheel Poses : Outport
  wires:
  conv_RotWheelRR/1(QuaternionVisu [rad]) -> Mux5/8
  conv_RotWheelRL/1(QuaternionVisu [rad]) -> Mux5/6
  conv_TransWheelRR/1(transVisu [m]) -> Mux5/7
  conv_TransWheelRL/1(transVisu [m]) -> Mux5/5
  conv_RotWheelFR/1(QuaternionVisu [rad]) -> Mux5/4
  conv_TransWheelFR/1(transVisu [m]) -> Mux5/3
  conv_RotWheelFL/1(QuaternionVisu [rad]) -> Mux5/2
  conv_TransWheelFL/1(transVisu [m]) -> Mux5/1
  Saturation/1 -> conv_TransWheelFL/1(transISO [m])
  Saturation8/1 -> conv_RotWheelFL/1(BryantISO [deg])
  Saturation2/1 -> conv_TransWheelFR/1(transISO [m])
  Saturation1/1 -> conv_RotWheelFR/1(BryantISO [deg])
  Saturation4/1 -> conv_TransWheelRL/1(transISO [m])
  Saturation3/1 -> conv_RotWheelRL/1(BryantISO [deg])
  Saturation6/1 -> conv_TransWheelRR/1(transISO [m])
  Saturation5/1 -> conv_RotWheelRR/1(BryantISO [deg])
  Mux5/1 -> Wheel Poses/1
  Mux2/1 -> Saturation3/1  "xyz rotation RL [deg]"
  Mux3/1 -> Saturation5/1  "xyz rotation RR [deg]"
  Mux/1 -> Saturation8/1  "xyz rotation FL [deg]"
  Mux1/1 -> Saturation1/1  "xyz rotation FR [deg]"
  Velocity [m/s]/1 -> omega=V/Rwheel/1
  omega=V/Rwheel/1 -> Radians to Degrees/1  "rotational speed [rad/s]"
  Steer Angle Rear [deg]/1 -> Mux2/3, Mux3/3  "rotz"
  Steer Angle Front [deg]/1 -> Mux/3, Mux1/3  "rotz"
  Constant4/1 -> Mux/1  "rotx"
  Constant5/1 -> Mux1/1  "rotx"
  Constant6/1 -> Mux2/1  "rotx"
  Constant7/1 -> Mux3/1  "rotx"
  Radians to Degrees/1 -> Discrete-Time Integrator/1
  Discrete-Time Integrator/1 -> Mux3/2, Mux2/2, Mux1/2, Mux/2  "roty"
  Disp FL [m]/1 -> Saturation/1
  Disp FR [m]/1 -> Saturation2/1
  Disp RL [m]/1 -> Saturation4/1
  Disp RR [m]/1 -> Saturation6/1

== system DvrSimKeybdGD_cs_old/Roewe_550_S_Sedan_1/SELF_Demux/compas converter ==
  rotz [rad] : Inport
  cart2compas : Subsystem
  rad2deg : Gain  Gain=180/pi
  heading [deg] : Outport
  wires:
  rad2deg/1 -> cart2compas/1(Angle [deg])
  rotz [rad]/1 -> rad2deg/1
  cart2compas/1(heading [deg]) -> heading [deg]/1

== system DvrSimKeybdGD_cs_old/Roewe_550_S_Sedan_1/Subsystem/TyreContact To Road Information ==
  TyreInfo_in : Inport
  Bus Selector3 : BusSelector  OutputSignals=TireFL.normal.x,TireFL.normal.y,TireFL.normal.z,TireFL.position.z,TireFR.normal.x,TireFR.normal.y,TireFR.normal.z,TireFR.position.z,TireRL.normal.x,TireRL.normal.y,TireRL.normal.z,TireRL.position.z,TireRR.normal.x,TireRR.normal.y,TireRR.normal.z,TireRR.position.z
  Contact To Road Information : Subsystem
  RoadSlopeAndZ_[FL;FR;RL;RR] : Outport
  wires:
  Bus Selector3/8 -> Contact To Road Information/8(" Pos_z_CP_CoorSys_E[FR]m]")  "<z>"
  Bus Selector3/7 -> Contact To Road Information/7(UnitVec_z_CP_CoorSys_E[FR][z])  "<z>"
  Contact To Road Information/1(RoadSlopeAndZ_[FL;FR;RL;RR]) -> RoadSlopeAndZ_[FL;FR;RL;RR]/1
  Bus Selector3/16 -> Contact To Road Information/16(" Pos_z_CP_CoorSys_E[RR]m]")  "<z>"
  Bus Selector3/15 -> Contact To Road Information/15(UnitVec_z_CP_CoorSys_E[RR][z])  "<z>"
  Bus Selector3/14 -> Contact To Road Information/14(UnitVec_z_CP_CoorSys_E[RR][y])  "<y>"
  Bus Selector3/13 -> Contact To Road Information/13(UnitVec_z_CP_CoorSys_E[RR][x])  "<x>"
  Bus Selector3/12 -> Contact To Road Information/12(" Pos_z_CP_CoorSys_E[RL]m]")  "<z>"
  Bus Selector3/11 -> Contact To Road Information/11(UnitVec_z_CP_CoorSys_E[RL][z])  "<z>"
  Bus Selector3/10 -> Contact To Road Information/10(UnitVec_z_CP_CoorSys_E[RL][y])  "<y>"
  Bus Selector3/9 -> Contact To Road Information/9(UnitVec_z_CP_CoorSys_E[RL][x])  "<x>"
  Bus Selector3/6 -> Contact To Road Information/6(UnitVec_z_CP_CoorSys_E[FR][y])  "<y>"
  Bus Selector3/5 -> Contact To Road Information/5(UnitVec_z_CP_CoorSys_E[FR][x])  "<x>"
  Bus Selector3/4 -> Contact To Road Information/4(" Pos_z_CP_CoorSys_E[FL]m]")  "<z>"
  Bus Selector3/3 -> Contact To Road Information/3(UnitVec_z_CP_CoorSys_E[FL][z])  "<z>"
  Bus Selector3/2 -> Contact To Road Information/2(UnitVec_z_CP_CoorSys_E[FL][y])  "<y>"
  Bus Selector3/1 -> Contact To Road Information/1(UnitVec_z_CP_CoorSys_E[FL][x])  "<x>"
  TyreInfo_in/1 -> Bus Selector3/1

== system DvrSimKeybdGD_cs_old/Roewe_550_S_Sedan_1/Subsystem1/CarSim2PreScanSTATE ==
  CarSim_In : Inport
  D2R : Gain  Gain=pi/180
  Demux : Demux  Outputs=[3 3 3 -1]
  Demux1 : Demux  Outputs=3
  Demux2 : Demux  Outputs=3
  Demux3 : Demux  Outputs=3
  Terminator : Terminator
  Transformation_SprungMassCarSim2PreScan : Subsystem
  km|h_to_m|s : Gain  Gain=1/3.6
  x [m] : Outport
  y [m] : Outport  Port=2
  z [m] : Outport  Port=3
  dx [m/s] : Outport  Port=4
  dy [m/s] : Outport  Port=5
  dz [m/s] : Outport  Port=6
  R [rad] : Outport  Port=7
  P [rad] : Outport  Port=8
  Y [rad] : Outport  Port=9
  wires:
  Demux/4 -> Terminator/1
  Demux3/3 -> Y [rad]/1
  Demux3/2 -> P [rad]/1
  Demux3/1 -> R [rad]/1
  Demux2/3 -> dz [m/s]/1
  Demux2/2 -> dy [m/s]/1
  Demux2/1 -> dx [m/s]/1
  Demux1/3 -> z [m]/1
  Demux1/2 -> y [m]/1
  Demux1/1 -> x [m]/1
  Transformation_SprungMassCarSim2PreScan/1(Out1) -> Demux1/1
  Demux/1 -> Transformation_SprungMassCarSim2PreScan/1(In1)
  CarSim_In/1 -> Demux/1
  km|h_to_m|s/1 -> Demux2/1
  Demux/2 -> km|h_to_m|s/1
  Demux/3 -> D2R/1
  D2R/1 -> Demux3/1
